simulink library "propertyLib"  (R2015a)
settings: Solver=ode45  StartTime=0.0  StopTime=10.0  RelTol=1e-3
undefined symbols (not defined in the file): mintspeed
libraries: sldvlib x20, simulink x7, propertyLib x2
settings Model: CovSFcnEnable=off  Creator=colosky  LastModifiedBy=colosky
settings DebuggingCC: SolverPrmCheckMsg=warning

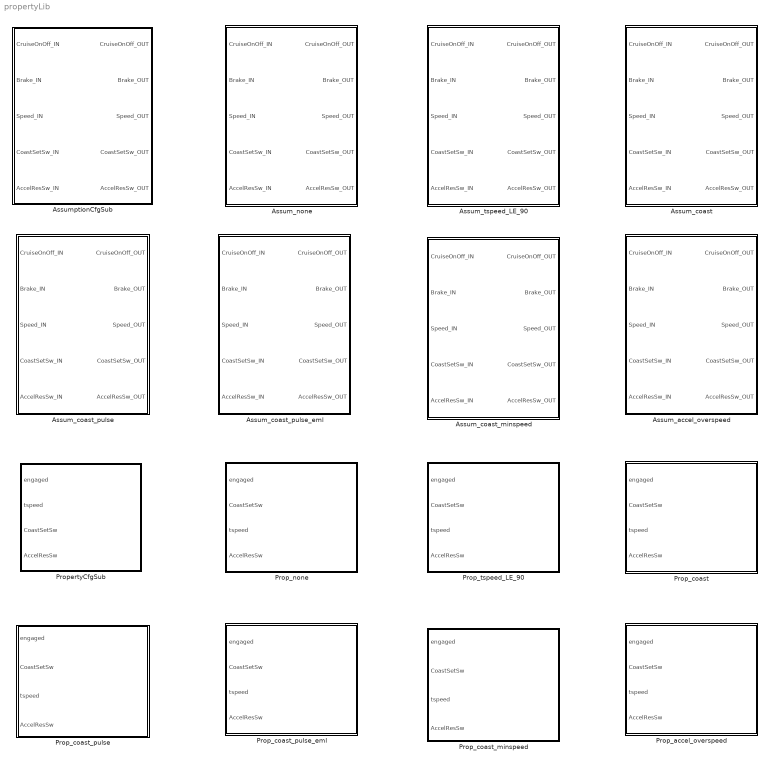
== system propertyLib ==
  Assum_accel_overspeed : Subsystem
  Assum_coast : Subsystem
  Assum_coast_minspeed : Subsystem
  Assum_coast_pulse : Subsystem
  Assum_coast_pulse_eml : Subsystem
  Assum_none : Subsystem
  Assum_tspeed_LE_90 : Subsystem
  AssumptionCfgSub : Subsystem  BlockChoice=Assum_tspeed_LE_90
      settings: TemplateBlock=self  MemberBlocks=Assum_accel_overspeed,Assum_coast,Assum_coast_minspeed,Assum_coast_pulse,Assum_coast_pulse_eml,Assum_none,Assum_tspeed_LE_90
  Prop_accel_overspeed : Subsystem
  Prop_coast : Subsystem
  Prop_coast_minspeed : Subsystem
  Prop_coast_pulse : Subsystem
  Prop_coast_pulse_eml : Subsystem
  Prop_none : Subsystem
  Prop_tspeed_LE_90 : Subsystem
  PropertyCfgSub : Subsystem  BlockChoice=Prop_none
      settings: TemplateBlock=self  MemberBlocks=Prop_accel_overspeed,Prop_coast,Prop_coast_minspeed,Prop_coast_pulse,Prop_coast_pulse_eml,Prop_none,Prop_tspeed_LE_90

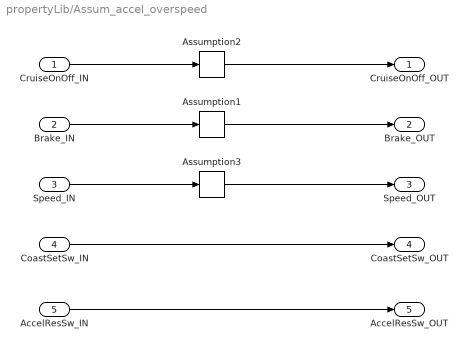
== system propertyLib/Assum_accel_overspeed ==
  CruiseOnOff_IN : Inport  OutDataTypeStr=boolean  PortDimensions=1
  Brake_IN : Inport  Port=2  OutDataTypeStr=boolean  PortDimensions=1
  Speed_IN : Inport  Port=3  OutDataTypeStr=uint8  PortDimensions=1
  CoastSetSw_IN : Inport  Port=4  OutDataTypeStr=boolean  PortDimensions=1
  AccelResSw_IN : Inport  Port=5  OutDataTypeStr=boolean  PortDimensions=1
  Assumption1 : sldvlib/Objectives and Constraints/Assumption  enabled=on  customAVTBlockType=Assumption  intervals=false  initial=off  dispValues=on  outEnabled=on
      settings: AttributesFormatString=%<intervals>
  Assumption2 : sldvlib/Objectives and Constraints/Assumption  enabled=on  customAVTBlockType=Assumption  intervals=true  initial=off  dispValues=on  outEnabled=on
      settings: AttributesFormatString=%<intervals>
  Assumption3 : sldvlib/Objectives and Constraints/Assumption  enabled=on  customAVTBlockType=Assumption  intervals={[88 Inf]}  initial=off  dispValues=on  outEnabled=on
      settings: AttributesFormatString=%<intervals>
  CruiseOnOff_OUT : Outport
  Brake_OUT : Outport  Port=2
  Speed_OUT : Outport  Port=3
  CoastSetSw_OUT : Outport  Port=4
  AccelResSw_OUT : Outport  Port=5
  wires:
  Speed_IN/1 -> Assumption3/1
  CoastSetSw_IN/1 -> CoastSetSw_OUT/1
  AccelResSw_IN/1 -> AccelResSw_OUT/1
  Brake_IN/1 -> Assumption1/1
  CruiseOnOff_IN/1 -> Assumption2/1
  Assumption2/1 -> CruiseOnOff_OUT/1
  Assumption1/1 -> Brake_OUT/1
  Assumption3/1 -> Speed_OUT/1

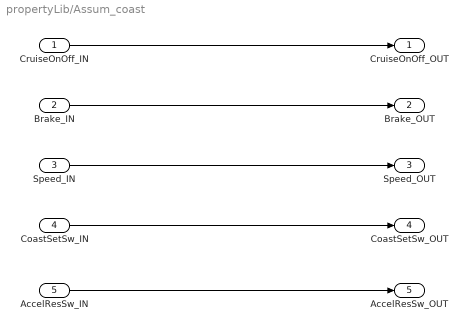
== system propertyLib/Assum_coast ==
  CruiseOnOff_IN : Inport  OutDataTypeStr=boolean  PortDimensions=1
  Brake_IN : Inport  Port=2  OutDataTypeStr=boolean  PortDimensions=1
  Speed_IN : Inport  Port=3  OutDataTypeStr=uint8  PortDimensions=1
  CoastSetSw_IN : Inport  Port=4  OutDataTypeStr=boolean  PortDimensions=1
  AccelResSw_IN : Inport  Port=5  OutDataTypeStr=boolean  PortDimensions=1
  CruiseOnOff_OUT : Outport
  Brake_OUT : Outport  Port=2
  Speed_OUT : Outport  Port=3
  CoastSetSw_OUT : Outport  Port=4
  AccelResSw_OUT : Outport  Port=5
  wires:
  CoastSetSw_IN/1 -> CoastSetSw_OUT/1
  Speed_IN/1 -> Speed_OUT/1
  CruiseOnOff_IN/1 -> CruiseOnOff_OUT/1
  Brake_IN/1 -> Brake_OUT/1
  AccelResSw_IN/1 -> AccelResSw_OUT/1

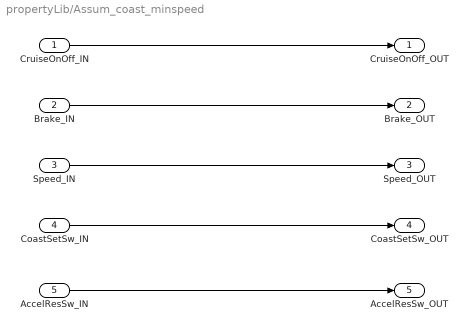
== system propertyLib/Assum_coast_minspeed ==
  CruiseOnOff_IN : Inport  OutDataTypeStr=boolean  PortDimensions=1
  Brake_IN : Inport  Port=2  OutDataTypeStr=boolean  PortDimensions=1
  Speed_IN : Inport  Port=3  OutDataTypeStr=uint8  PortDimensions=1
  CoastSetSw_IN : Inport  Port=4  OutDataTypeStr=boolean  PortDimensions=1
  AccelResSw_IN : Inport  Port=5  OutDataTypeStr=boolean  PortDimensions=1
  CruiseOnOff_OUT : Outport
  Brake_OUT : Outport  Port=2
  Speed_OUT : Outport  Port=3
  CoastSetSw_OUT : Outport  Port=4
  AccelResSw_OUT : Outport  Port=5
  wires:
  CoastSetSw_IN/1 -> CoastSetSw_OUT/1
  Speed_IN/1 -> Speed_OUT/1
  CruiseOnOff_IN/1 -> CruiseOnOff_OUT/1
  Brake_IN/1 -> Brake_OUT/1
  AccelResSw_IN/1 -> AccelResSw_OUT/1

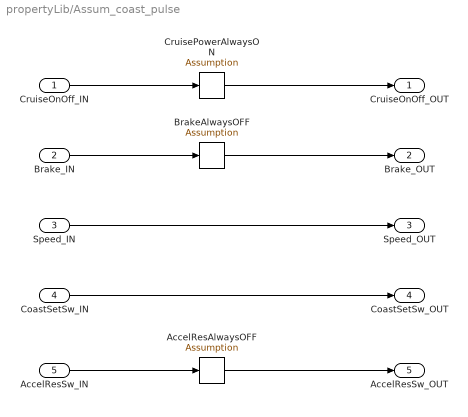
== system propertyLib/Assum_coast_pulse ==
  CruiseOnOff_IN : Inport  OutDataTypeStr=boolean  PortDimensions=1
  Brake_IN : Inport  Port=2  OutDataTypeStr=boolean  PortDimensions=1
  Speed_IN : Inport  Port=3  OutDataTypeStr=uint8  PortDimensions=1
  CoastSetSw_IN : Inport  Port=4  OutDataTypeStr=boolean  PortDimensions=1
  AccelResSw_IN : Inport  Port=5  OutDataTypeStr=boolean  PortDimensions=1
  AccelResAlwaysOFF : sldvlib/Objectives and Constraints/Assumption  enabled=on  customAVTBlockType=Assumption  intervals=false  initial=off  dispValues=on  outEnabled=on
      settings: AttributesFormatString=%<intervals>
  BrakeAlwaysOFF : sldvlib/Objectives and Constraints/Assumption  enabled=on  customAVTBlockType=Assumption  intervals=false  initial=off  dispValues=on  outEnabled=on
      settings: AttributesFormatString=%<intervals>
  CruisePowerAlwaysON : sldvlib/Objectives and Constraints/Assumption  enabled=on  customAVTBlockType=Assumption  intervals=true  initial=off  dispValues=on  outEnabled=on
      settings: AttributesFormatString=%<intervals>
  CruiseOnOff_OUT : Outport
  Brake_OUT : Outport  Port=2
  Speed_OUT : Outport  Port=3
  CoastSetSw_OUT : Outport  Port=4
  AccelResSw_OUT : Outport  Port=5
  wires:
  AccelResAlwaysOFF/1 -> AccelResSw_OUT/1
  BrakeAlwaysOFF/1 -> Brake_OUT/1
  CruisePowerAlwaysON/1 -> CruiseOnOff_OUT/1
  CruiseOnOff_IN/1 -> CruisePowerAlwaysON/1
  Brake_IN/1 -> BrakeAlwaysOFF/1
  Speed_IN/1 -> Speed_OUT/1
  AccelResSw_IN/1 -> AccelResAlwaysOFF/1
  CoastSetSw_IN/1 -> CoastSetSw_OUT/1

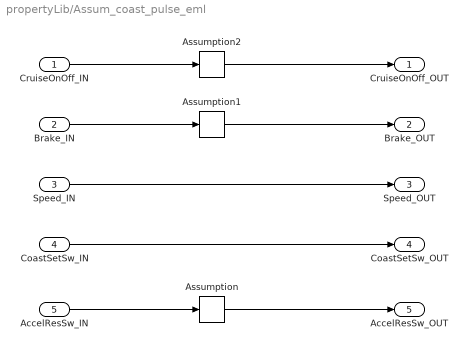
== system propertyLib/Assum_coast_pulse_eml ==
  CruiseOnOff_IN : Inport  OutDataTypeStr=boolean  PortDimensions=1
  Brake_IN : Inport  Port=2  OutDataTypeStr=boolean  PortDimensions=1
  Speed_IN : Inport  Port=3  OutDataTypeStr=uint8  PortDimensions=1
  CoastSetSw_IN : Inport  Port=4  OutDataTypeStr=boolean  PortDimensions=1
  AccelResSw_IN : Inport  Port=5  OutDataTypeStr=boolean  PortDimensions=1
  Assumption : sldvlib/Objectives and Constraints/Assumption  enabled=on  customAVTBlockType=Assumption  intervals=false  initial=off  dispValues=on  outEnabled=on
      settings: AttributesFormatString=%<intervals>
  Assumption1 : sldvlib/Objectives and Constraints/Assumption  enabled=on  customAVTBlockType=Assumption  intervals=false  initial=off  dispValues=on  outEnabled=on
      settings: AttributesFormatString=%<intervals>
  Assumption2 : sldvlib/Objectives and Constraints/Assumption  enabled=on  customAVTBlockType=Assumption  intervals=true  initial=off  dispValues=on  outEnabled=on
      settings: AttributesFormatString=%<intervals>
  CruiseOnOff_OUT : Outport
  Brake_OUT : Outport  Port=2
  Speed_OUT : Outport  Port=3
  CoastSetSw_OUT : Outport  Port=4
  AccelResSw_OUT : Outport  Port=5
  wires:
  CoastSetSw_IN/1 -> CoastSetSw_OUT/1
  AccelResSw_IN/1 -> Assumption/1
  Speed_IN/1 -> Speed_OUT/1
  Brake_IN/1 -> Assumption1/1
  CruiseOnOff_IN/1 -> Assumption2/1
  Assumption2/1 -> CruiseOnOff_OUT/1
  Assumption1/1 -> Brake_OUT/1
  Assumption/1 -> AccelResSw_OUT/1

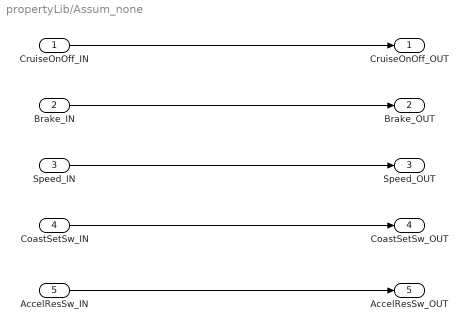
== system propertyLib/Assum_none ==
  CruiseOnOff_IN : Inport  OutDataTypeStr=boolean  PortDimensions=1
  Brake_IN : Inport  Port=2  OutDataTypeStr=boolean  PortDimensions=1
  Speed_IN : Inport  Port=3  OutDataTypeStr=uint8  PortDimensions=1
  CoastSetSw_IN : Inport  Port=4  OutDataTypeStr=boolean  PortDimensions=1
  AccelResSw_IN : Inport  Port=5  OutDataTypeStr=boolean  PortDimensions=1
  CruiseOnOff_OUT : Outport
  Brake_OUT : Outport  Port=2
  Speed_OUT : Outport  Port=3
  CoastSetSw_OUT : Outport  Port=4
  AccelResSw_OUT : Outport  Port=5
  wires:
  CoastSetSw_IN/1 -> CoastSetSw_OUT/1
  AccelResSw_IN/1 -> AccelResSw_OUT/1
  Speed_IN/1 -> Speed_OUT/1
  Brake_IN/1 -> Brake_OUT/1
  CruiseOnOff_IN/1 -> CruiseOnOff_OUT/1

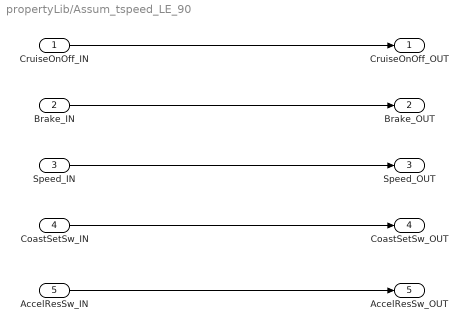
== system propertyLib/Assum_tspeed_LE_90 ==
  CruiseOnOff_IN : Inport  OutDataTypeStr=boolean  PortDimensions=1
  Brake_IN : Inport  Port=2  OutDataTypeStr=boolean  PortDimensions=1
  Speed_IN : Inport  Port=3  OutDataTypeStr=uint8  PortDimensions=1
  CoastSetSw_IN : Inport  Port=4  OutDataTypeStr=boolean  PortDimensions=1
  AccelResSw_IN : Inport  Port=5  OutDataTypeStr=boolean  PortDimensions=1
  CruiseOnOff_OUT : Outport
  Brake_OUT : Outport  Port=2
  Speed_OUT : Outport  Port=3
  CoastSetSw_OUT : Outport  Port=4
  AccelResSw_OUT : Outport  Port=5
  wires:
  CruiseOnOff_IN/1 -> CruiseOnOff_OUT/1
  Brake_IN/1 -> Brake_OUT/1
  AccelResSw_IN/1 -> AccelResSw_OUT/1
  CoastSetSw_IN/1 -> CoastSetSw_OUT/1
  Speed_IN/1 -> Speed_OUT/1

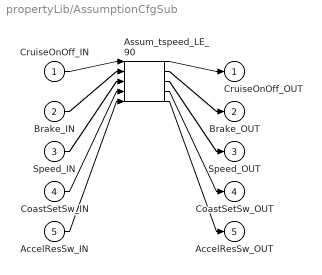
== system propertyLib/AssumptionCfgSub ==
  CruiseOnOff_IN : Inport
  Brake_IN : Inport  Port=2
  Speed_IN : Inport  Port=3
  CoastSetSw_IN : Inport  Port=4
  AccelResSw_IN : Inport  Port=5
  Assum_tspeed_LE_90 : propertyLib/Assum_tspeed_LE_90
  CruiseOnOff_OUT : Outport
  Brake_OUT : Outport  Port=2
  Speed_OUT : Outport  Port=3
  CoastSetSw_OUT : Outport  Port=4
  AccelResSw_OUT : Outport  Port=5
  wires:
  CruiseOnOff_IN/1 -> Assum_tspeed_LE_90/1
  Brake_IN/1 -> Assum_tspeed_LE_90/2
  Speed_IN/1 -> Assum_tspeed_LE_90/3
  CoastSetSw_IN/1 -> Assum_tspeed_LE_90/4
  AccelResSw_IN/1 -> Assum_tspeed_LE_90/5
  Assum_tspeed_LE_90/1 -> CruiseOnOff_OUT/1
  Assum_tspeed_LE_90/2 -> Brake_OUT/1
  Assum_tspeed_LE_90/3 -> Speed_OUT/1
  Assum_tspeed_LE_90/4 -> CoastSetSw_OUT/1
  Assum_tspeed_LE_90/5 -> AccelResSw_OUT/1

== system propertyLib/Prop_accel_overspeed ==
  engaged : Inport
  CoastSetSw : Inport  Port=2
  tspeed : Inport  Port=3
  AccelResSw : Inport  Port=4
  Compare To Constant : simulink/Logic and Bit Operations/Compare To Constant  relop=<=  const=95  OutDataTypeStr=boolean
  EngagedImplies : sldvlib/Verification Utilities/Implies
  Logical Operator2 : Logic  AllPortsSameDT=off  OutDataTypeStr=boolean
  Proof Objective : sldvlib/Objectives and Constraints/Proof Objective  enabled=on  customAVTBlockType=Proof Objective  intervals=true  dispValues=on  outEnabled=off  enableStopSim=off
      settings: AttributesFormatString=%<intervals>
  Terminator1 : Terminator
  wires:
  CoastSetSw/1 -> Terminator1/1
  tspeed/1 -> Compare To Constant/1
  Compare To Constant/1 -> EngagedImplies/2
  engaged/1 -> Logical Operator2/1
  AccelResSw/1 -> Logical Operator2/2
  Logical Operator2/1 -> EngagedImplies/1
  EngagedImplies/1 -> Proof Objective/1

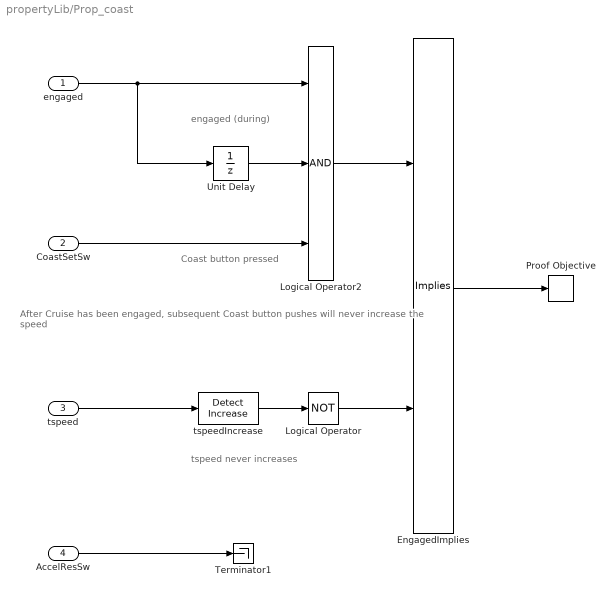
== system propertyLib/Prop_coast ==
  note: engaged (during)
  note: tspeed never increases
  note: Coast button pressed
  note: After Cruise has been engaged, subsequent Coast button pushes will never increase the speed
  engaged : Inport
  CoastSetSw : Inport  Port=2
  tspeed : Inport  Port=3
  AccelResSw : Inport  Port=4
  EngagedImplies : sldvlib/Verification Utilities/Implies
  Logical Operator : Logic  Operator=NOT  AllPortsSameDT=off  OutDataTypeStr=boolean
  Logical Operator2 : Logic  Inputs=3  AllPortsSameDT=off  OutDataTypeStr=boolean
  Proof Objective : sldvlib/Objectives and Constraints/Proof Objective  enabled=on  customAVTBlockType=Proof Objective  intervals=true  dispValues=on  outEnabled=off  enableStopSim=off
      settings: AttributesFormatString=%<intervals>
  Terminator1 : Terminator
  Unit Delay : UnitDelay  SampleTime=-1
  tspeedIncrease : simulink/Logic and Bit Operations/Detect Increase  vinit=0.0  InputProcessing=Inherited  OutDataTypeStr=boolean
  wires:
  Logical Operator2/1 -> EngagedImplies/1
  CoastSetSw/1 -> Logical Operator2/3
  Logical Operator/1 -> EngagedImplies/2
  engaged/1 -> Unit Delay/1, Logical Operator2/1
  AccelResSw/1 -> Terminator1/1
  Unit Delay/1 -> Logical Operator2/2
  tspeed/1 -> tspeedIncrease/1
  tspeedIncrease/1 -> Logical Operator/1
  EngagedImplies/1 -> Proof Objective/1

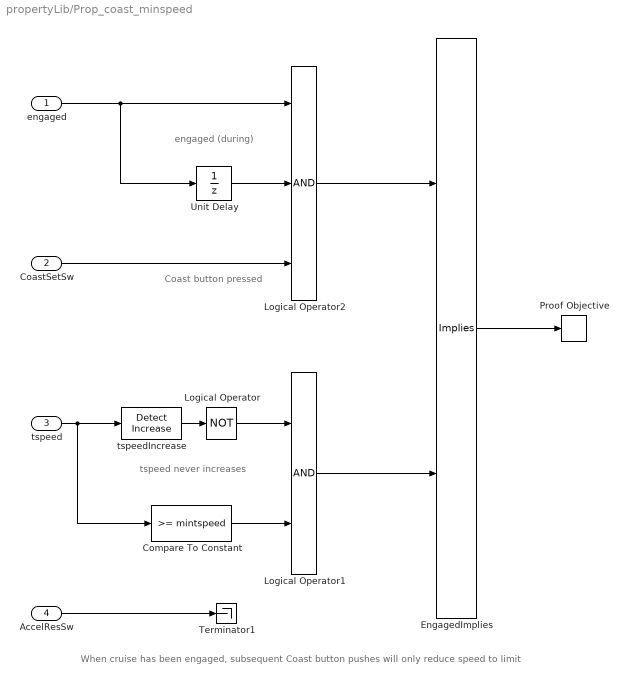
== system propertyLib/Prop_coast_minspeed ==
  note: engaged (during)
  note: tspeed never increases
  note: Coast button pressed
  note: When cruise has been engaged, subsequent Coast button pushes will only reduce speed to limit
  engaged : Inport
  CoastSetSw : Inport  Port=2
  tspeed : Inport  Port=3
  AccelResSw : Inport  Port=4
  Compare To Constant : simulink/Logic and Bit Operations/Compare To Constant  relop=>=  const=mintspeed  OutDataTypeStr=boolean
  EngagedImplies : sldvlib/Verification Utilities/Implies
  Logical Operator : Logic  Operator=NOT  AllPortsSameDT=off  OutDataTypeStr=boolean
  Logical Operator1 : Logic  AllPortsSameDT=off  OutDataTypeStr=boolean
  Logical Operator2 : Logic  Inputs=3  AllPortsSameDT=off  OutDataTypeStr=boolean
  Proof Objective : sldvlib/Objectives and Constraints/Proof Objective  enabled=on  customAVTBlockType=Proof Objective  intervals=true  dispValues=on  outEnabled=off  enableStopSim=off
      settings: AttributesFormatString=%<intervals>
  Terminator1 : Terminator
  Unit Delay : UnitDelay  SampleTime=-1
  tspeedIncrease : simulink/Logic and Bit Operations/Detect Increase  vinit=0.0  InputProcessing=Inherited  OutDataTypeStr=boolean
  wires:
  Logical Operator2/1 -> EngagedImplies/1
  CoastSetSw/1 -> Logical Operator2/3
  engaged/1 -> Unit Delay/1, Logical Operator2/1
  AccelResSw/1 -> Terminator1/1
  Unit Delay/1 -> Logical Operator2/2
  tspeed/1 -> Compare To Constant/1, tspeedIncrease/1
  tspeedIncrease/1 -> Logical Operator/1
  EngagedImplies/1 -> Proof Objective/1
  Logical Operator/1 -> Logical Operator1/1
  Compare To Constant/1 -> Logical Operator1/2
  Logical Operator1/1 -> EngagedImplies/2

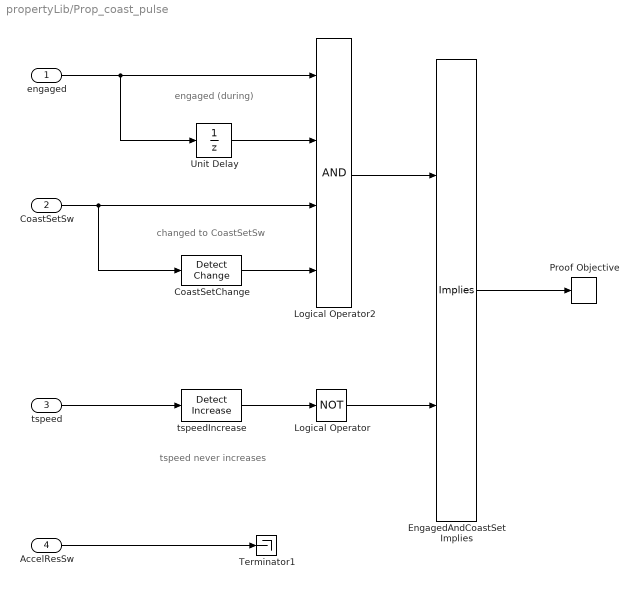
== system propertyLib/Prop_coast_pulse ==
  note: changed to CoastSetSw
  note: tspeed never increases
  note: engaged (during)
  engaged : Inport
  CoastSetSw : Inport  Port=2
  tspeed : Inport  Port=3
  AccelResSw : Inport  Port=4
  CoastSetChange : simulink/Logic and Bit Operations/Detect Change  vinit=0  InputProcessing=Inherited  OutDataTypeStr=boolean
  EngagedAndCoastSetImplies : sldvlib/Verification Utilities/Implies
  Logical Operator : Logic  Operator=NOT  AllPortsSameDT=off  OutDataTypeStr=boolean
  Logical Operator2 : Logic  Inputs=4  AllPortsSameDT=off  OutDataTypeStr=boolean
  Proof Objective : sldvlib/Objectives and Constraints/Proof Objective  enabled=on  customAVTBlockType=Proof Objective  intervals=true  dispValues=on  outEnabled=off  enableStopSim=off
      settings: AttributesFormatString=%<intervals>
  Terminator1 : Terminator
  Unit Delay : UnitDelay  SampleTime=-1
  tspeedIncrease : simulink/Logic and Bit Operations/Detect Increase  vinit=0.0  InputProcessing=Inherited  OutDataTypeStr=boolean
  wires:
  Logical Operator/1 -> EngagedAndCoastSetImplies/2
  CoastSetSw/1 -> Logical Operator2/3, CoastSetChange/1
  tspeed/1 -> tspeedIncrease/1
  Logical Operator2/1 -> EngagedAndCoastSetImplies/1
  AccelResSw/1 -> Terminator1/1
  tspeedIncrease/1 -> Logical Operator/1
  EngagedAndCoastSetImplies/1 -> Proof Objective/1
  engaged/1 -> Unit Delay/1, Logical Operator2/1
  Unit Delay/1 -> Logical Operator2/2
  CoastSetChange/1 -> Logical Operator2/4

== system propertyLib/Prop_coast_pulse_eml ==
  engaged : Inport
  CoastSetSw : Inport  Port=2
  tspeed : Inport  Port=3
  AccelResSw : Inport  Port=4
  MATLAB Function : MATLAB Function  TreatAsAtomicUnit=on
  Proof Objective : sldvlib/Objectives and Constraints/Proof Objective  enabled=on  customAVTBlockType=Proof Objective  intervals=true  dispValues=on  outEnabled=off  enableStopSim=off
      settings: AttributesFormatString=%<intervals>
  Terminator1 : Terminator
  wires:
  AccelResSw/1 -> Terminator1/1
  engaged/1 -> MATLAB Function/1(engaged)
  CoastSetSw/1 -> MATLAB Function/2(CoastSetSw)
  tspeed/1 -> MATLAB Function/3(tspeed)
  MATLAB Function/1(property) -> Proof Objective/1

== system propertyLib/Prop_none ==
  engaged : Inport
  CoastSetSw : Inport  Port=2
  tspeed : Inport  Port=3
  AccelResSw : Inport  Port=4
  Proof Objective : sldvlib/Objectives and Constraints/Proof Objective  enabled=on  customAVTBlockType=Proof Objective  intervals=true  dispValues=on  outEnabled=off  enableStopSim=off
      settings: AttributesFormatString=%<intervals>
  Terminator{,1..3} (4 alike) : Terminator
  trueProp : Constant  OutDataTypeStr=boolean
  wires:
  CoastSetSw/1 -> Terminator1/1
  tspeed/1 -> Terminator2/1
  engaged/1 -> Terminator/1
  AccelResSw/1 -> Terminator3/1
  trueProp/1 -> Proof Objective/1

== system propertyLib/Prop_tspeed_LE_90 ==
  engaged : Inport
  CoastSetSw : Inport  Port=2
  tspeed : Inport  Port=3
  AccelResSw : Inport  Port=4
  Compare To Constant : simulink/Logic and Bit Operations/Compare To Constant  relop=<=  const=90  OutDataTypeStr=boolean
  Proof Objective : sldvlib/Objectives and Constraints/Proof Objective  enabled=on  customAVTBlockType=Proof Objective  intervals=true  dispValues=on  outEnabled=off  enableStopSim=off
      settings: AttributesFormatString=%<intervals>
  Terminator : Terminator
  Terminator1 : Terminator
  Terminator2 : Terminator
  wires:
  engaged/1 -> Terminator/1
  tspeed/1 -> Compare To Constant/1
  CoastSetSw/1 -> Terminator1/1
  AccelResSw/1 -> Terminator2/1
  Compare To Constant/1 -> Proof Objective/1

== system propertyLib/PropertyCfgSub ==
  engaged : Inport
  tspeed : Inport  Port=2
  CoastSetSw : Inport  Port=3
  AccelResSw : Inport  Port=4
  Prop_none : propertyLib/Prop_none
  wires:
  engaged/1 -> Prop_none/1
  CoastSetSw/1 -> Prop_none/2
  tspeed/1 -> Prop_none/3
  AccelResSw/1 -> Prop_none/4

== matlab function propertyLib/Prop_coast_pulse_eml/MATLAB Function ==
  data: engaged input; property output; CoastSetSw input; tspeed input
function property = Prop_coast_pulse(engaged,CoastSetSw,tspeed)
%#codegen
persistent  engagedLast;
persistent  CoastSetSwLast;
persistent  tspeedLast;

% initialize Last(s) one time
if isempty(engagedLast)
    engagedLast = false; 
    CoastSetSwLast = false; 
    tspeedLast = uint8(0); 
end

% at least last two times engaged
engagedCond = engaged && engagedLast;

% pulsing CoastSetSw
CoastSetSwCond = CoastSetSw && ~CoastSetSwLast;

% tspeed never increase
tspeedCond = tspeed<=tspeedLast;

% property
property = true;
if engagedCond && CoastSetSwCond 
    property = tspeedCond;
end

% update Last(s)
engagedLast = engaged; 
CoastSetSwLast = CoastSetSw; 
tspeedLast = tspeed;
